simulink model "CaseStudyII_9_Bus"  (R2020a)
settings: Solver=FixedStepAuto  StartTime=0.0  StopTime=Tend  FixedStep=T_s_power  MaxStep=5.0E-5  RelTol=1e-3
values from neighbouring files (symbols this model uses):
  B_s46 = b_s46*Cb    (= 9.5071761847e-07)    [Data_CaseStudyI.m]    (also in Data_CaseStudyII.m; Data_InitialSystem.m)
  B_s54 = b_s54*Cb    (= 1.05902722057e-06)    [Data_CaseStudyI.m]    (also in Data_CaseStudyII.m; Data_InitialSystem.m)
  B_s69 = b_s69*Cb    (= 2.15415764185e-06)    [Data_CaseStudyI.m]    (also in Data_CaseStudyII.m; Data_InitialSystem.m)
  B_s75 = b_s75*Cb    (= 1.84126323577e-06)    [Data_CaseStudyI.m]    (also in Data_CaseStudyII.m; Data_InitialSystem.m)
  B_s87 = b_s87*Cb    (= 8.96562817417e-07)    [Data_CaseStudyI.m]    (also in Data_CaseStudyII.m; Data_InitialSystem.m)
  B_s98 = b_s98*Cb    (= 1.25759482443e-06)    [Data_CaseStudyI.m]    (also in Data_CaseStudyII.m; Data_InitialSystem.m)
  C_dc_DVPP_1_2 = 0.008*(n_DVPP_1_2)    (= 0.8)    [Data_CaseStudyI.m]    (also in Data_CaseStudyII.m)
  C_dc_DVPP_1_3 = 0.008*(n_DVPP_1_3)    (= 0.4)    [Data_CaseStudyI.m]    (also in Data_CaseStudyII.m)
  C_dc_DVPP_3_1 = 0.008*(n_DVPP_3_1)    (= 1.128)    [Data_CaseStudyII.m]
  C_dc_DVPP_3_2 = 0.008*(n_DVPP_3_2)    (= 0.848)    [Data_CaseStudyII.m]
  C_dc_DVPP_3_3 = 0.008*(n_DVPP_3_3)    (= 1.28)    [Data_CaseStudyII.m]
  Dp_DVPP_3_pu = 1/dp_DVPP_3    (= 33.3333333333)    [Data_CaseStudyII.m]
  Dq1_DVPP_3_pu = 100    [Data_CaseStudyII.m]
  fb = 50    [Data_CaseStudyI.m]    (also in Data_CaseStudyII.m; Data_InitialSystem.m)
  HGov_dyn = HGov_delay*H_tr_droop    [Data_CaseStudyI.m]    (also in Data_CaseStudyII.m; Data_InitialSystem.m)
  HTurb_tot = H_water_way    [Data_CaseStudyI.m]    (also in Data_CaseStudyII.m; Data_InitialSystem.m)
  I_m_DVPP_1_2 = 2/3*Sb_DVPP_1_2/V_m_DVPP_1_2    [Data_CaseStudyI.m]    (also in Data_CaseStudyII.m)
  I_m_DVPP_1_3 = 2/3*Sb_DVPP_1_3/V_m_DVPP_1_3    [Data_CaseStudyI.m]    (also in Data_CaseStudyII.m)
  I_m_DVPP_3_1 = 2/3*Sb_DVPP_3_1/V_m_DVPP_3_1    [Data_CaseStudyII.m]
  I_m_DVPP_3_2 = 2/3*Sb_DVPP_3_2/V_m_DVPP_3_2    [Data_CaseStudyII.m]
  I_m_DVPP_3_3 = 2/3*Sb_DVPP_3_3/V_m_DVPP_3_3    [Data_CaseStudyII.m]
  i_star_max = 1.3    [Data_CaseStudyI.m]    (also in Data_CaseStudyII.m)
  iabc_DVPP_1_2_0 = T0*idq0_DVPP_1_2    [Data_CaseStudyI.m]    (also in Data_CaseStudyII.m)
  iabc_DVPP_1_3_0 = T0*idq0_DVPP_1_3    [Data_CaseStudyI.m]    (also in Data_CaseStudyII.m)
  iabc_DVPP_3_1_0 = T0*idq0_DVPP_3_1    [Data_CaseStudyII.m]
  iabc_DVPP_3_2_0 = T0*idq0_DVPP_3_2    [Data_CaseStudyII.m]
  iabc_DVPP_3_3_0 = T0*idq0_DVPP_3_3    [Data_CaseStudyII.m]
  K2_DVPP_1 = [-0.0221795494247 -1.60799665656 0.160449825826 -2.94803557381 -11.8081988371 -9.75170960256 0.00463021906909 -49.1667298155]    [ControlGains_DVPP1.mat]
  K3_DVPP_1 = [-0.0591512752956 -1.61493903379 -27.2946107927 -16.2119211358 -14.3657419818 2.05688388773 -2.27328406162 0.146700393037 -150.920793597]    [ControlGains_DVPP1.mat]
  k_dc_DVPP_1_2 = eta_DVPP_1_2/(Vdc_n_DVPP_1_2*m_p_DVPP_1_2)    [Data_CaseStudyI.m]    (also in Data_CaseStudyII.m)
  k_dc_DVPP_1_3 = eta_DVPP_1_3/(Vdc_n_DVPP_1_3*m_p_DVPP_1_3)    [Data_CaseStudyI.m]    (also in Data_CaseStudyII.m)
  k_dc_DVPP_3_1 = eta_DVPP_3_1/(Vdc_n_DVPP_3_1*m_p_DVPP_3_1)    [Data_CaseStudyII.m]
  k_dc_DVPP_3_2 = eta_DVPP_3_2/(Vdc_n_DVPP_3_2*m_p_DVPP_3_2)    [Data_CaseStudyII.m]
  k_dc_DVPP_3_3 = eta_DVPP_3_3/(Vdc_n_DVPP_3_3*m_p_DVPP_3_3)    [Data_CaseStudyII.m]
  ki_i_pu = 1.19    [Data_CaseStudyI.m]    (also in Data_CaseStudyII.m)
  ki_pll = 1700    [Data_CaseStudyI.m]    (also in Data_CaseStudyII.m)
  ki_q_pu = 0.005    [Data_CaseStudyI.m]    (also in Data_CaseStudyII.m)
  kp_i_pu = 0.73    [Data_CaseStudyI.m]    (also in Data_CaseStudyII.m)
  kp_pll = 150    [Data_CaseStudyI.m]    (also in Data_CaseStudyII.m)
  kp_q_pu = 0.05    [Data_CaseStudyI.m]    (also in Data_CaseStudyII.m)
  L1_DVPP_1_2_pu = 0.0186/m_DVPP_1_2    (= 0.000372)    [Data_CaseStudyI.m]    (also in Data_CaseStudyII.m)
  L1_DVPP_1_3_pu = 0.0186/m_DVPP_1_3    (= 0.000744)    [Data_CaseStudyI.m]    (also in Data_CaseStudyII.m)
  L1_DVPP_3_1_pu = 0.0186/m_DVPP_3_1    (= 0.000263829787234)    [Data_CaseStudyII.m]
  L1_DVPP_3_2_pu = 0.0186/m_DVPP_3_2    (= 0.000350943396226)    [Data_CaseStudyII.m]
  L1_DVPP_3_3_pu = 0.0186/m_DVPP_3_3    (= 0.0002325)    [Data_CaseStudyII.m]
  l1_MVHV1 = 0    [Data_CaseStudyI.m]    (also in Data_CaseStudyII.m; Data_InitialSystem.m)
  l1_MVHV2 = 0    [Data_CaseStudyI.m]    (also in Data_CaseStudyII.m; Data_InitialSystem.m)
  l1_MVHV3 = 0    [Data_CaseStudyI.m]    (also in Data_CaseStudyII.m; Data_InitialSystem.m)
  L2_DVPP_1_2_pu = L1_DVPP_1_2_pu    (= 0.000372)    [Data_CaseStudyI.m]    (also in Data_CaseStudyII.m)
  L2_DVPP_1_3_pu = L1_DVPP_1_3_pu    (= 0.000744)    [Data_CaseStudyI.m]    (also in Data_CaseStudyII.m)
  L2_DVPP_3_1_pu = L1_DVPP_3_1_pu    (= 0.000263829787234)    [Data_CaseStudyII.m]
  L2_DVPP_3_2_pu = L1_DVPP_3_2_pu    (= 0.000350943396226)    [Data_CaseStudyII.m]
  L2_DVPP_3_3_pu = L1_DVPP_3_3_pu    (= 0.0002325)    [Data_CaseStudyII.m]
  l2_MVHV1 = l_s14    (= 0.0576)    [Data_CaseStudyI.m]    (also in Data_CaseStudyII.m; Data_InitialSystem.m)
  l2_MVHV2 = l_s72    (= 0.0625)    [Data_CaseStudyI.m]    (also in Data_CaseStudyII.m; Data_InitialSystem.m)
  l2_MVHV3 = l_s39    (= 0.0586)    [Data_CaseStudyI.m]    (also in Data_CaseStudyII.m; Data_InitialSystem.m)
  l_f_DVPP_1_2 = L_f_DVPP_1_2*w_b/Zb_DVPP_1_2    [Data_CaseStudyI.m]    (also in Data_CaseStudyII.m)
  L_f_DVPP_1_2 = (1/(n_DVPP_1_2))*600*10^-6    (= 6e-06)    [Data_CaseStudyI.m]    (also in Data_CaseStudyII.m)
  l_f_DVPP_1_3 = L_f_DVPP_1_3*w_b/Zb_DVPP_1_3    [Data_CaseStudyI.m]    (also in Data_CaseStudyII.m)
  L_f_DVPP_1_3 = (1/(n_DVPP_1_3))*600*10^-6    (= 1.2e-05)    [Data_CaseStudyI.m]    (also in Data_CaseStudyII.m)
  l_f_DVPP_3_1 = L_f_DVPP_3_1*w_b/Zb_DVPP_3_1    [Data_CaseStudyII.m]
  L_f_DVPP_3_1 = (1/(n_DVPP_3_1))*600*10^-6    (= 4.25531914894e-06)    [Data_CaseStudyII.m]
  l_f_DVPP_3_2 = L_f_DVPP_3_2*w_b/Zb_DVPP_3_2    [Data_CaseStudyII.m]
  L_f_DVPP_3_2 = (1/(n_DVPP_3_2))*600*10^-6    (= 5.66037735849e-06)    [Data_CaseStudyII.m]
  l_f_DVPP_3_3 = L_f_DVPP_3_3*w_b/Zb_DVPP_3_3    [Data_CaseStudyII.m]
  L_f_DVPP_3_3 = (1/(n_DVPP_3_3))*600*10^-6    (= 3.75e-06)    [Data_CaseStudyII.m]
  L_s46 = l_s46*Lb    (= 0.154915055408)    [Data_CaseStudyI.m]    (also in Data_CaseStudyII.m; Data_InitialSystem.m)
  L_s54 = l_s54*Lb    (= 0.143128040323)    [Data_CaseStudyI.m]    (also in Data_CaseStudyII.m; Data_InitialSystem.m)
  L_s69 = l_s69*Lb    (= 0.286256080645)    [Data_CaseStudyI.m]    (also in Data_CaseStudyII.m; Data_InitialSystem.m)
  L_s75 = l_s75*Lb    (= 0.271101346964)    [Data_CaseStudyI.m]    (also in Data_CaseStudyII.m; Data_InitialSystem.m)
  L_s87 = l_s87*Lb    (= 0.12123786945)    [Data_CaseStudyI.m]    (also in Data_CaseStudyII.m; Data_InitialSystem.m)
  L_s98 = l_s98*Lb    (= 0.16973301723)    [Data_CaseStudyI.m]    (also in Data_CaseStudyII.m; Data_InitialSystem.m)
  LPV_K1_DVPP_3 = [0.014519129833 -1.24253756746e-17 -0.00331576987938 -1.41950397655e-17 -0.00331577010739 -1.6423216922e-19 0.0145191298795 1.47256053017e-18 1.92456501739e-17 0.00968260817745 7.5102914291e-19 0.0096826081765 ... (80 elements, 8x10)]    [ControlGains_DVPP3_LPV.mat]
  LPV_K2_DVPP_3 = [0.0299413265511 -2.72480441208e-16 -0.00563144274341 -6.63344905835e-17 -0.00563144273182 -1.08918556426e-16 0.0299413268326 -1.32404731664e-16 -4.78559537004e-17 -0.00914230292149 -8.50409089014e-21 -0.00914230292147 ... (80 elements, 8x10)]    [ControlGains_DVPP3_LPV.mat]
  LPV_K3_DVPP_3 = [-0.0173301370849 5.00398589077e-17 -0.0636125194304 3.31757376688e-17 -0.0636125164794 5.41726806116e-17 -0.017330137145 2.43427565927e-17 -0.0400570975704 -5.68753124238e-17 -0.0574012283733 2.45717741258e-17 ... (192 elements, 16x12)]    [ControlGains_DVPP3_LPV.mat]
  Mp_DVPP_3_pu = 13    [Data_CaseStudyII.m]
  P_L = pL*Sb    (= 300000000)    [Data_CaseStudyI.m]    (also in Data_CaseStudyII.m; Data_InitialSystem.m)
  p_set_bus1 = P_set_bus1/SbSG1    (= 0.731707317073)    [Data_CaseStudyI.m]    (also in Data_CaseStudyII.m; Data_InitialSystem.m)
  p_set_bus2 = P_set_bus2/SbSG2    (= 0.756707317073)    [Data_CaseStudyI.m]    (also in Data_CaseStudyII.m; Data_InitialSystem.m)
  Pb_DVPP_3_1 = 37e6    (= 37000000)    [Data_CaseStudyII.m]
  Pb_DVPP_3_2 = 28e6    (= 28000000)    [Data_CaseStudyII.m]
  Pb_DVPP_3_3 = 0e6    (= 0)    [Data_CaseStudyII.m]
  pset_DVPP_1_1 = P_set_bus1/SbSG1    (= 0.731707317073)    [Data_CaseStudyI.m]    (also in Data_CaseStudyII.m)
  pset_DVPP_1_2 = 0    [Data_CaseStudyI.m]    (also in Data_CaseStudyII.m)
  pset_DVPP_1_3 = 0    [Data_CaseStudyI.m]    (also in Data_CaseStudyII.m)
  pset_DVPP_3_1 = (0.6*P_set_bus3)/Sb_DVPP_3_1    (= 0.398546964193)    [Data_CaseStudyII.m]
  pset_DVPP_3_2 = (0.4*P_set_bus3)/Sb_DVPP_3_2    (= 0.353428439945)    [Data_CaseStudyII.m]
  pset_DVPP_3_3 = 0    [Data_CaseStudyII.m]
  Q_L = qL*Sb    (= 82500000)    [Data_CaseStudyI.m]    (also in Data_CaseStudyII.m; Data_InitialSystem.m)
  qset_DVPP_1_2 = 0    [Data_CaseStudyI.m]    (also in Data_CaseStudyII.m)
  qset_DVPP_1_3 = 0    [Data_CaseStudyI.m]    (also in Data_CaseStudyII.m)
  qset_DVPP_3_1 = 0    [Data_CaseStudyII.m]
  qset_DVPP_3_2 = 0    [Data_CaseStudyII.m]
  qset_DVPP_3_3 = 0    [Data_CaseStudyII.m]
  R1_DVPP_1_2_pu = 0.00734/m_DVPP_1_2    (= 0.0001468)    [Data_CaseStudyI.m]    (also in Data_CaseStudyII.m)
  R1_DVPP_1_3_pu = 0.00734/m_DVPP_1_3    (= 0.0002936)    [Data_CaseStudyI.m]    (also in Data_CaseStudyII.m)
  R1_DVPP_3_1_pu = 0.00734/m_DVPP_3_1    (= 0.000104113475177)    [Data_CaseStudyII.m]
  R1_DVPP_3_2_pu = 0.00734/m_DVPP_3_2    (= 0.000138490566038)    [Data_CaseStudyII.m]
  R1_DVPP_3_3_pu = 0.00734/m_DVPP_3_3    (= 9.175e-05)    [Data_CaseStudyII.m]
  r1_MVHV1 = 1e-6    (= 1e-06)    [Data_CaseStudyI.m]    (also in Data_CaseStudyII.m; Data_InitialSystem.m)
  r1_MVHV2 = 1e-6    (= 1e-06)    [Data_CaseStudyI.m]    (also in Data_CaseStudyII.m; Data_InitialSystem.m)
  r1_MVHV3 = 1e-6    (= 1e-06)    [Data_CaseStudyI.m]    (also in Data_CaseStudyII.m; Data_InitialSystem.m)
  R2_DVPP_1_2_pu = R1_DVPP_1_2_pu    (= 0.0001468)    [Data_CaseStudyI.m]    (also in Data_CaseStudyII.m)
  R2_DVPP_1_3_pu = R1_DVPP_1_3_pu    (= 0.0002936)    [Data_CaseStudyI.m]    (also in Data_CaseStudyII.m)
  R2_DVPP_3_1_pu = R1_DVPP_3_1_pu    (= 0.000104113475177)    [Data_CaseStudyII.m]
  R2_DVPP_3_2_pu = R1_DVPP_3_2_pu    (= 0.000138490566038)    [Data_CaseStudyII.m]
  R2_DVPP_3_3_pu = R1_DVPP_3_3_pu    (= 9.175e-05)    [Data_CaseStudyII.m]
  r2_MVHV1 = 1e-6    (= 1e-06)    [Data_CaseStudyI.m]    (also in Data_CaseStudyII.m; Data_InitialSystem.m)
  r2_MVHV2 = 1e-6    (= 1e-06)    [Data_CaseStudyI.m]    (also in Data_CaseStudyII.m; Data_InitialSystem.m)
  r2_MVHV3 = 1e-6    (= 1e-06)    [Data_CaseStudyI.m]    (also in Data_CaseStudyII.m; Data_InitialSystem.m)
  R_dc_DVPP_1_2 = (Vdc_n_DVPP_1_2/(0.05*(Sb_DVPP_1_2)/Vdc_n_DVPP_1_2))    [Data_CaseStudyI.m]    (also in Data_CaseStudyII.m)
  R_dc_DVPP_1_3 = (Vdc_n_DVPP_1_3/(0.05*(Sb_DVPP_1_3)/Vdc_n_DVPP_1_3))    [Data_CaseStudyI.m]    (also in Data_CaseStudyII.m)
  R_dc_DVPP_3_1 = (Vdc_n_DVPP_3_1/(0.05*(Sb_DVPP_3_1)/Vdc_n_DVPP_3_1))    [Data_CaseStudyII.m]
  R_dc_DVPP_3_2 = (Vdc_n_DVPP_3_2/(0.05*(Sb_DVPP_3_2)/Vdc_n_DVPP_3_2))    [Data_CaseStudyII.m]
  R_dc_DVPP_3_3 = (Vdc_n_DVPP_3_3/(0.05*(Sb_DVPP_3_3)/Vdc_n_DVPP_3_3))    [Data_CaseStudyII.m]
  r_f_DVPP_1_2 = R_f_DVPP_1_2/Zb_DVPP_1_2    [Data_CaseStudyI.m]    (also in Data_CaseStudyII.m)
  R_f_DVPP_1_2 = 0.02/n_DVPP_1_2    (= 0.0002)    [Data_CaseStudyI.m]    (also in Data_CaseStudyII.m)
  r_f_DVPP_1_3 = R_f_DVPP_1_3/Zb_DVPP_1_3    [Data_CaseStudyI.m]    (also in Data_CaseStudyII.m)
  R_f_DVPP_1_3 = 0.02/n_DVPP_1_3    (= 0.0004)    [Data_CaseStudyI.m]    (also in Data_CaseStudyII.m)
  r_f_DVPP_3_1 = R_f_DVPP_3_1/Zb_DVPP_3_1    [Data_CaseStudyII.m]
  ... (+104 more)
undefined symbols (not defined in the file or in its folder): A, B, C, Continuous, Dd, Efd0, gcbh, i_dc, Ka, Kf, p2set, SbSM2, sps_rtmsupport, spsST1AModel, Ta, Tb, Tb1, Tc, Tc1, Tf, VA0, VAmax, VAmin, VImax, VImin, VRmax, VRmin
libraries: powerlib x95, powerlib_meascontrol x41, cstblocks x15, sps_avr x1, simulink_extras x1, simulink x1
(part 2 of 5)

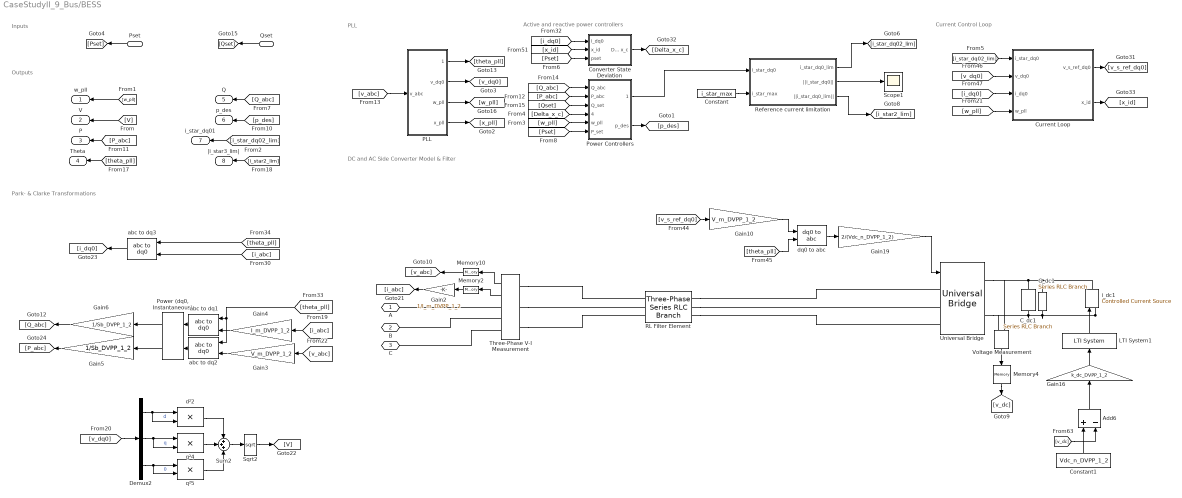
== system CaseStudyII_9_Bus/BESS ==
  note: Inputs
  note: Active and reactive power controllers
  note: PLL
  note: Outputs
  note: Current Control Loop
  note: Park- & Clarke Transformations
  note: DC and AC Side Converter Model & Filter
  Qset : Inport
  Pset : Inport  Port=2
  Add6 : Sum  Inputs=+-
  C_dc1 : powerlib/Elements/Series RLC Branch  LConnTagsString=__new0  RConnTagsString=__new0  BranchType=C  Resistance=1  Inductance=1e-3  SetiL0=off  InitialCurrent=0  Capacitance=C_dc_DVPP_1_2  Setx0=off  InitialVoltage=Vdc_n  Measurements=None
  Constant : Constant  Value=i_star_max
  Constant1 : Constant  Value=Vdc_n_DVPP_1_2
  Converter State Deviation : Subsystem
  Current Loop : Subsystem  AncestorBlock=Library/Grid-Forming Converter Controlled by Droop Control /Current Loop
  Demux2 : Demux  Outputs=3
  G_dc1 : powerlib/Elements/Series RLC Branch  LConnTagsString=__new0  RConnTagsString=__new0  BranchType=R  Resistance=R_dc_DVPP_1_2  Inductance=1e-3  SetiL0=off  InitialCurrent=0  Capacitance=1e-6  Setx0=off  InitialVoltage=0  Measurements=None
  Gain10 : Gain  Gain=V_m_DVPP_1_2
  Gain16 : Gain  Gain=k_dc_DVPP_1_2
  Gain19 : Gain  Gain=2/(Vdc_n_DVPP_1_2)
  Gain2 : Gain  Gain=1/I_m_DVPP_1_2
  Gain3 : Gain  Gain=V_m_DVPP_1_2
  Gain4 : Gain  Gain=I_m_DVPP_1_2
  Gain5 : Gain  Gain=1/Sb_DVPP_1_2
  Gain6 : Gain  Gain=1/Sb_DVPP_1_2
  LTI System1 : cstblocks/LTI System  sys=tf(1,[tau_dc_DVPP_1_2 1])  IC=[]
  Memory10 : Memory  InitialCondition=[vabc_DVPP_1_2_0_pu(1), vabc_DVPP_1_2_0_pu(2), vabc_DVPP_1_2_0_pu(3)]
  Memory2 : Memory  InitialCondition=[iabc_DVPP_1_2_0(1), iabc_DVPP_1_2_0(2), iabc_DVPP_1_2_0(3)]
  Memory4 : Memory
  PLL : Subsystem
  "Power (dq0, Instantaneous)" : powerlib_meascontrol/Measurements/Power (dq0, Instantaneous)
      settings: SourceProductBaseCode=PS
  Power Controllers : Subsystem
  RL Filter Element : powerlib/Elements/Three-Phase Series RLC Branch  LConnTagsString=A|B|C  RConnTagsString=A|B|C  BranchType=RL  Resistance=R_f_DVPP_1_2  Inductance=L_f_DVPP_1_2  Capacitance=0  Measurements=Branch currents
  Reference current limitation : Subsystem
  Scope1 : Scope
  Sqrt2 : Sqrt  SaturateOnIntegerOverflow=on
  Sum2 : Sum  Inputs=+++  InputSameDT=on  SaturateOnIntegerOverflow=on  OutDataTypeStr=Inherit: Same as first input
  Three-Phase V-I Measurement : powerlib/Measurements/Three-Phase V-I Measurement  VoltageMeasurement=phase-to-ground  SetLabelV=off  LabelV=Vabc  Vpu=on  VpuLL=off  CurrentMeasurement=yes  SetLabelI=off  LabelI=Iabc  Ipu=off  Pbase=Sb_conv  Vbase=VbLV_DVPP_1_2  OutputType=Complex  PhasorSimulation=off  PSBequivalent=0
  Universal Bridge : powerlib/Power Electronics/Universal Bridge  Arms=3  SnubberResistance=1e5  SnubberCapacitance=inf  Device=Average-model based VSC  Ron=1e-3  Lon=0  ForwardVoltages="[  0  0  ]"  ForwardVoltage=0  GTOparameters=[ 10e-6 , 20e-6 ]  IGBTparameters=[ 1e-6 , 2e-6 ]  Measurements=None  Measurements_2=None  converterType=Rectifier
  Voltage Measurement : powerlib/Measurements/Voltage Measurement  PhasorSimulation=off  OutputType=Complex  PSBequivalent=0
  abc to dq1 : powerlib_meascontrol/Transformations/abc to dq0  Alignment=90 degrees behind phase A axis
  abc to dq2 : powerlib_meascontrol/Transformations/abc to dq0  Alignment=90 degrees behind phase A axis
  abc to dq3 : powerlib_meascontrol/Transformations/abc to dq0  Alignment=90 degrees behind phase A axis
  dq0 to abc : powerlib_meascontrol/Transformations/dq0 to abc  Alignment=90 degrees behind phase A axis
  d²2 : Product  InputSameDT=on  RndMeth=Zero  SaturateOnIntegerOverflow=on  OutDataTypeStr=Inherit: Same as first input
  i_dc1 : powerlib/Electrical Sources/Controlled Current Source  Initialize=off  Source_Type=DC  Amplitude=i_dc  Phase=0  Frequency=0  Measurements=None
  q²4 : Product  InputSameDT=on  RndMeth=Zero  SaturateOnIntegerOverflow=on  OutDataTypeStr=Inherit: Same as first input
  q²5 : Product  InputSameDT=on  RndMeth=Zero  SaturateOnIntegerOverflow=on  OutDataTypeStr=Inherit: Same as first input
  A : PMIOPort  Side=Right
  B : PMIOPort  Port=2  Side=Right
  C : PMIOPort  Port=3  Side=Right
  w_pll : Outport  VectorParamsAs1DForOutWhenUnconnected=off
  V : Outport  Port=2  VectorParamsAs1DForOutWhenUnconnected=off
  P : Outport  Port=3  VectorParamsAs1DForOutWhenUnconnected=off
  Theta : Outport  Port=4  VectorParamsAs1DForOutWhenUnconnected=off
  Q : Outport  Port=5  VectorParamsAs1DForOutWhenUnconnected=off
  p_des : Outport  Port=6  VectorParamsAs1DForOutWhenUnconnected=off
  i_star_dq01 : Outport  Port=7  VectorParamsAs1DForOutWhenUnconnected=off
  |i_star3_lim| : Outport  Port=8  VectorParamsAs1DForOutWhenUnconnected=off
  wires:
  PLL/4(x_pll) -> [x_pll]
  [v_abc] -> PLL/1(v_abc)
  [i_star_dq02_lim] -> i_star_dq01/1
  PLL/2(v_dq0) -> [v_dq0]
  [p_des] -> p_des/1
  PLL/1(theta_pll) -> [theta_pll]
  PLL/3(w_pll) -> [w_pll]
  [V] -> V/1
  [w_pll] -> w_pll/1
  [theta_pll] -> Theta/1
  Power Controllers/2(p_des) -> [p_des]
  Power Controllers/1(i_star_dq0) -> Reference current limitation/1(i_star_dq0)
  [Q_abc] -> Q/1
  Qset/1 -> [Qset]
  [P_abc] -> P/1
  Constant/1 -> Reference current limitation/2(i_star_max)
  Reference current limitation/2(||i_star_dq0||) -> Scope1/1
  [i_star2_lim] -> |i_star3_lim|/1
  [w_pll] -> Current Loop/4(w_pll)
  [i_dq0] -> Current Loop/3(i_dq0)
  Reference current limitation/1(i_star_dq0_lim) -> [i_star_dq02_lim]
  [v_dq0] -> Current Loop/2(v_dq0)
  [v_dq0] -> Demux2/1
  Sum2/1 -> Sqrt2/1
  [i_abc] -> Gain4/1
  Demux2/3 -> q²5/2, q²5/1  "0"
  Demux2/1 -> d²2/1, d²2/2  "d"
  abc to dq1/1 -> "Power (dq0, Instantaneous)"/2
  Three-Phase V-I Measurement/1 -> Memory10/1
  Gain5/1 -> [P_abc]
  Gain4/1 -> abc to dq1/1
  Gain3/1 -> abc to dq2/1
  q²4/1 -> Sum2/2
  Gain6/1 -> [Q_abc]
  Gain19/1 -> Universal Bridge/1
  Add6/1 -> Gain16/1
  [v_abc] -> Gain3/1
  [theta_pll] -> abc to dq3/2
  abc to dq3/1 -> [i_dq0]
  Voltage Measurement/1 -> Memory4/1
  d²2/1 -> Sum2/1
  [theta_pll] -> abc to dq2/2, abc to dq1/2
  dq0 to abc/1 -> Gain19/1
  Memory10/1 -> [v_abc]
  "Power (dq0, Instantaneous)"/2 -> Gain6/1
  Sqrt2/1 -> [V]
  "Power (dq0, Instantaneous)"/1 -> Gain5/1
  Demux2/2 -> q²4/1, q²4/2  "q"
  [v_dc] -> Add6/2
  q²5/1 -> Sum2/3
  abc to dq2/1 -> "Power (dq0, Instantaneous)"/1
  Memory4/1 -> [v_dc]
  LTI System1/1 -> i_dc1/1
  Gain10/1 -> dq0 to abc/1
  [theta_pll] -> dq0 to abc/2
  [i_abc] -> abc to dq3/1
  [v_s_ref_dq0] -> Gain10/1
  Gain16/1 -> LTI System1/1
  Constant1/1 -> Add6/1
  Converter State Deviation/1(Delta x_c) -> [Delta_x_c]
  Current Loop/2(x_id) -> [x_id]
  Current Loop/1(v_s_ref_dq0) -> [v_s_ref_dq0]
  [P_abc] -> Power Controllers/2(P_abc)
  [Delta_x_c] -> Power Controllers/4(Delta x_c)
  [Q_abc] -> Power Controllers/1(Q_abc)
  [Qset] -> Power Controllers/3(Q_set)
  [x_id] -> Converter State Deviation/2(x_id)
  [i_dq0] -> Converter State Deviation/1(i_dq0)
  Reference current limitation/3(||i_star_dq0_lim||) -> [i_star2_lim]
  [i_star_dq02_lim] -> Current Loop/1(i_star_dq0)
  [w_pll] -> Power Controllers/5(w_pll)
  [Pset] -> Converter State Deviation/3(pset)
  Pset/1 -> [Pset]
  [Pset] -> Power Controllers/6(P_set)
  Gain2/1 -> [i_abc]
  Memory2/1 -> Gain2/1
  Three-Phase V-I Measurement/2 -> Memory2/1
  connections:
  i_dc1/LConn1 -- G_dc1/RConn1 -- Voltage Measurement/LConn2 -- Universal Bridge/RConn2 -- C_dc1/RConn1
  i_dc1/RConn1 -- G_dc1/LConn1 -- Voltage Measurement/LConn1 -- Universal Bridge/RConn1 -- C_dc1/LConn1
  RL Filter Element/RConn3 -- Universal Bridge/LConn3
  RL Filter Element/RConn2 -- Universal Bridge/LConn2
  RL Filter Element/RConn1 -- Universal Bridge/LConn1
  Three-Phase V-I Measurement/LConn1 -- RL Filter Element/LConn1
  Three-Phase V-I Measurement/LConn2 -- RL Filter Element/LConn2
  Three-Phase V-I Measurement/LConn3 -- RL Filter Element/LConn3
  Three-Phase V-I Measurement/RConn1 -- A/RConn1
  Three-Phase V-I Measurement/RConn2 -- B/RConn1
  Three-Phase V-I Measurement/RConn3 -- C/RConn1

== system CaseStudyII_9_Bus/DVPP Operator  ==
  pmax_1 : Inport
  pmax_2 : Inport  Port=2
  Add : Sum
  Constant : Constant  Value=Sb_DVPP_3_1
  Constant1 : Constant  Value=Sb_DVPP_3_2
  Constant2 : Constant  Value=Sb_DVPP_3_3
  Constant3 : Constant  Value=Pb_DVPP_3_3
  Divide : Product  Inputs=*/
  Divide1 : Product  Inputs=/*
  MATLAB Function : MATLAB Function  TreatAsAtomicUnit=on
  theta1_p : Outport
  theta2_p : Outport  Port=2
  theta1_q : Outport  Port=3
  theta2_q : Outport  Port=4
  theta3_q : Outport  Port=5
  wires:
  pmax_2/1 -> Add/2, MATLAB Function/5(P2), Divide1/2
  pmax_1/1 -> Divide/1, MATLAB Function/4(P1), Add/1
  Add/1 -> Divide1/1, Divide/2
  Divide1/1 -> theta2_p/1
  Divide/1 -> theta1_p/1
  Constant/1 -> MATLAB Function/1(S1)
  Constant1/1 -> MATLAB Function/2(S2)
  Constant2/1 -> MATLAB Function/3(S3)
  Constant3/1 -> MATLAB Function/6(P3)
  MATLAB Function/1(theta1_q) -> theta1_q/1
  MATLAB Function/2(theta2_q) -> theta2_q/1
  MATLAB Function/3(theta3_q) -> theta3_q/1

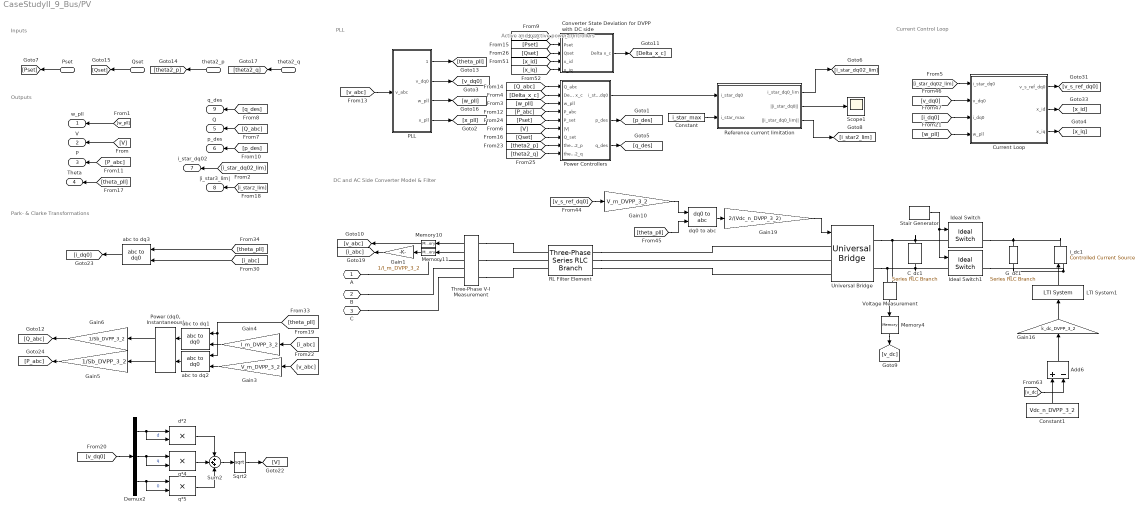
== system CaseStudyII_9_Bus/PV ==
  note: PLL
  note: Park- & Clarke Transformations
  note: Outputs
  note: Active and reactive power controllers
  note: Current Control Loop
  note: DC and AC Side Converter Model & Filter
  note: Inputs
  Pset : Inport
  Qset : Inport  Port=2
  theta2_p : Inport  Port=3
  theta2_q : Inport  Port=4
  Add6 : Sum  Inputs=+-
  C_dc1 : powerlib/Elements/Series RLC Branch  LConnTagsString=__new0  RConnTagsString=__new0  BranchType=C  Resistance=1  Inductance=1e-3  SetiL0=off  InitialCurrent=0  Capacitance=C_dc_DVPP_3_2  Setx0=off  InitialVoltage=Vdc_n  Measurements=None
  Constant : Constant  Value=i_star_max
  Constant1 : Constant  Value=Vdc_n_DVPP_3_2
  Converter State Deviation for DVPP with DC side : Subsystem
  Current Loop : Subsystem  AncestorBlock=Library/Grid-Forming Converter Controlled by Droop Control /Current Loop
  Demux2 : Demux  Outputs=3
  G_dc1 : powerlib/Elements/Series RLC Branch  LConnTagsString=__new0  RConnTagsString=__new0  BranchType=R  Resistance=R_dc_DVPP_3_2  Inductance=1e-3  SetiL0=off  InitialCurrent=0  Capacitance=1e-6  Setx0=off  InitialVoltage=0  Measurements=None
  Gain1 : Gain  Gain=1/I_m_DVPP_3_2
  Gain10 : Gain  Gain=V_m_DVPP_3_2
  Gain16 : Gain  Gain=k_dc_DVPP_3_2
  Gain19 : Gain  Gain=2/(Vdc_n_DVPP_3_2)
  Gain3 : Gain  Gain=V_m_DVPP_3_2
  Gain4 : Gain  Gain=I_m_DVPP_3_2
  Gain5 : Gain  Gain=1/Sb_DVPP_3_2
  Gain6 : Gain  Gain=1/Sb_DVPP_3_2
  Ideal Switch : powerlib/Power Electronics/Ideal Switch  Ron=0.001  Lon=0  IC=1  Rs=1e10  Cs=Inf  Measurements=on
  Ideal Switch1 : powerlib/Power Electronics/Ideal Switch  Ron=0.001  Lon=0  IC=1  Rs=1e10  Cs=Inf  Measurements=on
  LTI System1 : cstblocks/LTI System  sys=tf(1,[tau_dc_DVPP_3_2 1])  IC=[]
  Memory10 : Memory  InitialCondition=[vabc_DVPP_3_2_0_pu(1), vabc_DVPP_3_2_0_pu(2), vabc_DVPP_3_2_0_pu(3)]
  Memory11 : Memory  InitialCondition=[iabc_DVPP_3_2_0(1), iabc_DVPP_3_2_0(2), iabc_DVPP_3_2_0(3)]
  Memory4 : Memory
  PLL : Subsystem
  "Power (dq0, Instantaneous)" : powerlib_meascontrol/Measurements/Power (dq0, Instantaneous)
      settings: SourceProductBaseCode=PS
  Power Controllers : Subsystem
  RL Filter Element : powerlib/Elements/Three-Phase Series RLC Branch  LConnTagsString=A|B|C  RConnTagsString=A|B|C  BranchType=RL  Resistance=R_f_DVPP_3_2  Inductance=L_f_DVPP_3_2  Capacitance=0  Measurements=Branch currents
  Reference current limitation : Subsystem
  Scope1 : Scope
  Sqrt2 : Sqrt  SaturateOnIntegerOverflow=on
  Stair Generator : powerlib_meascontrol/Pulse & Signal Generators/Stair Generator  t=[0 T_cloud]  e=[1 0]  Ts=0
      settings: SourceProductBaseCode=MT,PS
  Sum2 : Sum  Inputs=+++  InputSameDT=on  SaturateOnIntegerOverflow=on  OutDataTypeStr=Inherit: Same as first input
  Three-Phase V-I Measurement : powerlib/Measurements/Three-Phase V-I Measurement  VoltageMeasurement=phase-to-ground  SetLabelV=off  LabelV=Vabc  Vpu=on  VpuLL=off  CurrentMeasurement=yes  SetLabelI=off  LabelI=Iabc  Ipu=off  Pbase=Sb_conv  Vbase=VbLV_DVPP_3_2  OutputType=Complex  PhasorSimulation=off  PSBequivalent=0
  Universal Bridge : powerlib/Power Electronics/Universal Bridge  Arms=3  SnubberResistance=1e5  SnubberCapacitance=inf  Device=Average-model based VSC  Ron=1e-3  Lon=0  ForwardVoltages="[  0  0  ]"  ForwardVoltage=0  GTOparameters=[ 10e-6 , 20e-6 ]  IGBTparameters=[ 1e-6 , 2e-6 ]  Measurements=None  Measurements_2=None  converterType=Rectifier
  Voltage Measurement : powerlib/Measurements/Voltage Measurement  PhasorSimulation=off  OutputType=Complex  PSBequivalent=0
  abc to dq1 : powerlib_meascontrol/Transformations/abc to dq0  Alignment=90 degrees behind phase A axis
  abc to dq2 : powerlib_meascontrol/Transformations/abc to dq0  Alignment=90 degrees behind phase A axis
  abc to dq3 : powerlib_meascontrol/Transformations/abc to dq0  Alignment=90 degrees behind phase A axis
  dq0 to abc : powerlib_meascontrol/Transformations/dq0 to abc  Alignment=90 degrees behind phase A axis
  d²2 : Product  InputSameDT=on  RndMeth=Zero  SaturateOnIntegerOverflow=on  OutDataTypeStr=Inherit: Same as first input
  i_dc1 : powerlib/Electrical Sources/Controlled Current Source  Initialize=off  Source_Type=DC  Amplitude=i_dc  Phase=0  Frequency=0  Measurements=None
  q²4 : Product  InputSameDT=on  RndMeth=Zero  SaturateOnIntegerOverflow=on  OutDataTypeStr=Inherit: Same as first input
  q²5 : Product  InputSameDT=on  RndMeth=Zero  SaturateOnIntegerOverflow=on  OutDataTypeStr=Inherit: Same as first input
  A : PMIOPort  Side=Right
  B : PMIOPort  Port=2  Side=Right
  C : PMIOPort  Port=3  Side=Right
  w_pll : Outport  VectorParamsAs1DForOutWhenUnconnected=off
  V : Outport  Port=2  VectorParamsAs1DForOutWhenUnconnected=off
  P : Outport  Port=3  VectorParamsAs1DForOutWhenUnconnected=off
  Theta : Outport  Port=4  VectorParamsAs1DForOutWhenUnconnected=off
  Q : Outport  Port=5  VectorParamsAs1DForOutWhenUnconnected=off
  p_des : Outport  Port=6  VectorParamsAs1DForOutWhenUnconnected=off
  i_star_dq02 : Outport  Port=7  VectorParamsAs1DForOutWhenUnconnected=off
  |i_star3_lim| : Outport  Port=8  VectorParamsAs1DForOutWhenUnconnected=off
  q_des : Outport  Port=9  VectorParamsAs1DForOutWhenUnconnected=off
  wires:
  [q_des] -> q_des/1
  [v_s_ref_dq0] -> Gain10/1
  Reference current limitation/3(||i_star_dq0_lim||) -> [i_star2_lim]
  [v_dq0] -> Demux2/1
  Three-Phase V-I Measurement/1 -> Memory10/1
  Voltage Measurement/1 -> Memory4/1
  [theta_pll] -> Theta/1
  [P_abc] -> P/1
  Memory11/1 -> Gain1/1
  [i_star_dq02_lim] -> Current Loop/1(i_star_dq0)
  Power Controllers/3(q_des) -> [q_des]
  Current Loop/3(x_iq) -> [x_iq]
  [Delta_x_c] -> Power Controllers/2(Delta x_c)
  Memory4/1 -> [v_dc]
  [v_dq0] -> Current Loop/2(v_dq0)
  Power Controllers/1(i_star_dq0) -> Reference current limitation/1(i_star_dq0)
  [V] -> V/1
  [w_pll] -> w_pll/1
  Current Loop/2(x_id) -> [x_id]
  [i_dq0] -> Current Loop/3(i_dq0)
  Gain1/1 -> [i_abc]
  [i_abc] -> Gain4/1
  PLL/1(theta_pll) -> [theta_pll]
  [v_abc] -> Gain3/1
  Gain5/1 -> [P_abc]
  Gain6/1 -> [Q_abc]
  Sum2/1 -> Sqrt2/1
  d²2/1 -> Sum2/1
  Gain10/1 -> dq0 to abc/1
  [i_star_dq02_lim] -> i_star_dq02/1
  Demux2/3 -> q²5/2, q²5/1  "0"
  dq0 to abc/1 -> Gain19/1
  q²5/1 -> Sum2/3
  LTI System1/1 -> i_dc1/1
  Add6/1 -> Gain16/1
  [i_star2_lim] -> |i_star3_lim|/1
  [Q_abc] -> Power Controllers/1(Q_abc)
  "Power (dq0, Instantaneous)"/2 -> Gain6/1
  [v_dc] -> Add6/2
  abc to dq2/1 -> "Power (dq0, Instantaneous)"/1
  [V] -> Power Controllers/6(|V|)
  "Power (dq0, Instantaneous)"/1 -> Gain5/1
  [i_abc] -> abc to dq3/1
  [theta_pll] -> abc to dq2/2, abc to dq1/2
  Gain16/1 -> LTI System1/1
  [theta_pll] -> dq0 to abc/2
  Sqrt2/1 -> [V]
  [v_abc] -> PLL/1(v_abc)
  [w_pll] -> Current Loop/4(w_pll)
  abc to dq3/1 -> [i_dq0]
  Constant1/1 -> Add6/1
  Gain19/1 -> Universal Bridge/1
  [Q_abc] -> Q/1
  Current Loop/1(v_s_ref_dq0) -> [v_s_ref_dq0]
  [theta_pll] -> abc to dq3/2
  [P_abc] -> Power Controllers/4(P_abc)
  Demux2/1 -> d²2/1, d²2/2  "d"
  Reference current limitation/1(i_star_dq0_lim) -> [i_star_dq02_lim]
  Reference current limitation/2(||i_star_dq0||) -> Scope1/1
  Gain3/1 -> abc to dq2/1
  Constant/1 -> Reference current limitation/2(i_star_max)
  abc to dq1/1 -> "Power (dq0, Instantaneous)"/2
  Demux2/2 -> q²4/1, q²4/2  "q"
  q²4/1 -> Sum2/2
  PLL/4(x_pll) -> [x_pll]
  PLL/2(v_dq0) -> [v_dq0]
  PLL/3(w_pll) -> [w_pll]
  Gain4/1 -> abc to dq1/1
  Memory10/1 -> [v_abc]
  Three-Phase V-I Measurement/2 -> Memory11/1
  [Pset] -> Power Controllers/5(P_set)
  Power Controllers/2(p_des) -> [p_des]
  [p_des] -> p_des/1
  [w_pll] -> Power Controllers/3(w_pll)
  Converter State Deviation for DVPP with DC side/1(Delta x_c) -> [Delta_x_c]
  [x_id] -> Converter State Deviation for DVPP with DC side/4(x_id)
  [x_iq] -> Converter State Deviation for DVPP with DC side/5(x_iq)
  [Qset] -> Converter State Deviation for DVPP with DC side/3(Qset)
  [Pset] -> Converter State Deviation for DVPP with DC side/2(Pset)
  [i_dq0] -> Converter State Deviation for DVPP with DC side/1(i_dq0)
  [Qset] -> Power Controllers/7(Q_set)
  Qset/1 -> [Qset]
  theta2_q/1 -> [theta2_q]
  Pset/1 -> [Pset]
  theta2_p/1 -> [theta2_p]
  [theta2_p] -> Power Controllers/8(theta2_p)
  [theta2_q] -> Power Controllers/9(theta2_q)
  Stair Generator/1 -> Ideal Switch1/1, Ideal Switch/1
  connections:
  i_dc1/RConn1 -- G_dc1/LConn1 -- Ideal Switch/RConn1
  i_dc1/LConn1 -- Ideal Switch1/RConn1 -- G_dc1/RConn1
  B/RConn1 -- Three-Phase V-I Measurement/RConn2
  Three-Phase V-I Measurement/LConn3 -- RL Filter Element/LConn3
  RL Filter Element/RConn1 -- Universal Bridge/LConn1
  Three-Phase V-I Measurement/LConn1 -- RL Filter Element/LConn1
  RL Filter Element/RConn2 -- Universal Bridge/LConn2
  A/RConn1 -- Three-Phase V-I Measurement/RConn1
  C/RConn1 -- Three-Phase V-I Measurement/RConn3
  Three-Phase V-I Measurement/LConn2 -- RL Filter Element/LConn2
  RL Filter Element/RConn3 -- Universal Bridge/LConn3
  Universal Bridge/RConn2 -- Ideal Switch1/LConn1 -- C_dc1/RConn1 -- Voltage Measurement/LConn2
  Voltage Measurement/LConn1 -- Universal Bridge/RConn1 -- C_dc1/LConn1 -- Ideal Switch/LConn1

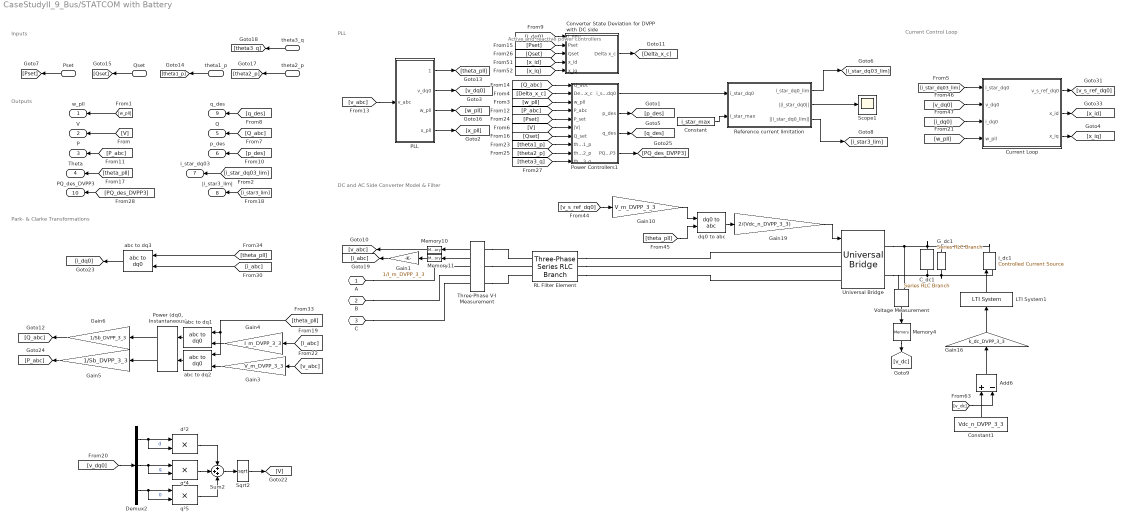
== system CaseStudyII_9_Bus/STATCOM with Battery ==
  note: Current Control Loop
  note: Park- & Clarke Transformations
  note: Outputs
  note: DC and AC Side Converter Model & Filter
  note: Active and reactive power controllers
  note: PLL
  note: Inputs
  Pset : Inport
  Qset : Inport  Port=2
  theta1_p : Inport  Port=3
  theta2_p : Inport  Port=4
  theta3_q : Inport  Port=5
  Add6 : Sum  Inputs=+-
  C_dc1 : powerlib/Elements/Series RLC Branch  LConnTagsString=__new0  RConnTagsString=__new0  BranchType=C  Resistance=1  Inductance=1e-3  SetiL0=off  InitialCurrent=0  Capacitance=C_dc_DVPP_3_3  Setx0=off  InitialVoltage=Vdc_n  Measurements=None
  Constant : Constant  Value=i_star_max
  Constant1 : Constant  Value=Vdc_n_DVPP_3_3
  Converter State Deviation for DVPP with DC side : Subsystem
  Current Loop : Subsystem  AncestorBlock=Library/Grid-Forming Converter Controlled by Droop Control /Current Loop
  Demux2 : Demux  Outputs=3
  G_dc1 : powerlib/Elements/Series RLC Branch  LConnTagsString=__new0  RConnTagsString=__new0  BranchType=R  Resistance=R_dc_DVPP_3_3  Inductance=1e-3  SetiL0=off  InitialCurrent=0  Capacitance=1e-6  Setx0=off  InitialVoltage=0  Measurements=None
  Gain1 : Gain  Gain=1/I_m_DVPP_3_3
  Gain10 : Gain  Gain=V_m_DVPP_3_3
  Gain16 : Gain  Gain=k_dc_DVPP_3_3
  Gain19 : Gain  Gain=2/(Vdc_n_DVPP_3_3)
  Gain3 : Gain  Gain=V_m_DVPP_3_3
  Gain4 : Gain  Gain=I_m_DVPP_3_3
  Gain5 : Gain  Gain=1/Sb_DVPP_3_3
  Gain6 : Gain  Gain=1/Sb_DVPP_3_3
  LTI System1 : cstblocks/LTI System  sys=tf(1,[tau_dc_DVPP_3_3 1])  IC=[]
  Memory10 : Memory  InitialCondition=[vabc_DVPP_3_3_0_pu(1), vabc_DVPP_3_3_0_pu(2), vabc_DVPP_3_3_0_pu(3)]
  Memory11 : Memory  InitialCondition=[iabc_DVPP_3_3_0(1), iabc_DVPP_3_3_0(2), iabc_DVPP_3_3_0(3)]
  Memory4 : Memory
  PLL : Subsystem
  "Power (dq0, Instantaneous)" : powerlib_meascontrol/Measurements/Power (dq0, Instantaneous)
      settings: SourceProductBaseCode=PS
  Power Controllers1 : Subsystem
  RL Filter Element : powerlib/Elements/Three-Phase Series RLC Branch  LConnTagsString=A|B|C  RConnTagsString=A|B|C  BranchType=RL  Resistance=R_f_DVPP_3_3  Inductance=L_f_DVPP_3_3  Capacitance=0  Measurements=Branch currents
  Reference current limitation : Subsystem
  Scope1 : Scope
  Sqrt2 : Sqrt  SaturateOnIntegerOverflow=on
  Sum2 : Sum  Inputs=+++  InputSameDT=on  SaturateOnIntegerOverflow=on  OutDataTypeStr=Inherit: Same as first input
  Three-Phase V-I Measurement : powerlib/Measurements/Three-Phase V-I Measurement  VoltageMeasurement=phase-to-ground  SetLabelV=off  LabelV=Vabc  Vpu=on  VpuLL=off  CurrentMeasurement=yes  SetLabelI=off  LabelI=Iabc  Ipu=off  Pbase=Sb_conv  Vbase=VbLV_DVPP_3_3  OutputType=Complex  PhasorSimulation=off  PSBequivalent=0
  Universal Bridge : powerlib/Power Electronics/Universal Bridge  Arms=3  SnubberResistance=1e5  SnubberCapacitance=inf  Device=Average-model based VSC  Ron=1e-3  Lon=0  ForwardVoltages="[  0  0  ]"  ForwardVoltage=0  GTOparameters=[ 10e-6 , 20e-6 ]  IGBTparameters=[ 1e-6 , 2e-6 ]  Measurements=None  Measurements_2=None  converterType=Rectifier
  Voltage Measurement : powerlib/Measurements/Voltage Measurement  PhasorSimulation=off  OutputType=Complex  PSBequivalent=0
  abc to dq1 : powerlib_meascontrol/Transformations/abc to dq0  Alignment=90 degrees behind phase A axis
  abc to dq2 : powerlib_meascontrol/Transformations/abc to dq0  Alignment=90 degrees behind phase A axis
  abc to dq3 : powerlib_meascontrol/Transformations/abc to dq0  Alignment=90 degrees behind phase A axis
  dq0 to abc : powerlib_meascontrol/Transformations/dq0 to abc  Alignment=90 degrees behind phase A axis
  d²2 : Product  InputSameDT=on  RndMeth=Zero  SaturateOnIntegerOverflow=on  OutDataTypeStr=Inherit: Same as first input
  i_dc1 : powerlib/Electrical Sources/Controlled Current Source  Initialize=off  Source_Type=DC  Amplitude=i_dc  Phase=0  Frequency=0  Measurements=None
  q²4 : Product  InputSameDT=on  RndMeth=Zero  SaturateOnIntegerOverflow=on  OutDataTypeStr=Inherit: Same as first input
  q²5 : Product  InputSameDT=on  RndMeth=Zero  SaturateOnIntegerOverflow=on  OutDataTypeStr=Inherit: Same as first input
  A : PMIOPort  Side=Right
  B : PMIOPort  Port=2  Side=Right
  C : PMIOPort  Port=3  Side=Right
  w_pll : Outport  VectorParamsAs1DForOutWhenUnconnected=off
  V : Outport  Port=2  VectorParamsAs1DForOutWhenUnconnected=off
  P : Outport  Port=3  VectorParamsAs1DForOutWhenUnconnected=off
  Theta : Outport  Port=4  VectorParamsAs1DForOutWhenUnconnected=off
  Q : Outport  Port=5  VectorParamsAs1DForOutWhenUnconnected=off
  p_des : Outport  Port=6  VectorParamsAs1DForOutWhenUnconnected=off
  i_star_dq03 : Outport  Port=7  VectorParamsAs1DForOutWhenUnconnected=off
  |i_star3_lim| : Outport  Port=8  VectorParamsAs1DForOutWhenUnconnected=off
  q_des : Outport  Port=9  VectorParamsAs1DForOutWhenUnconnected=off
  PQ_des_DVPP3 : Outport  Port=10  VectorParamsAs1DForOutWhenUnconnected=off
  wires:
  [p_des] -> p_des/1
  Memory10/1 -> [v_abc]
  [Pset] -> Power Controllers1/5(P_set)
  PLL/3(w_pll) -> [w_pll]
  PLL/2(v_dq0) -> [v_dq0]
  Demux2/2 -> q²4/1, q²4/2  "q"
  q²4/1 -> Sum2/2
  abc to dq1/1 -> "Power (dq0, Instantaneous)"/2
  Gain3/1 -> abc to dq2/1
  Reference current limitation/2(||i_star_dq0||) -> Scope1/1
  [P_abc] -> Power Controllers1/4(P_abc)
  [w_pll] -> Power Controllers1/3(w_pll)
  Demux2/1 -> d²2/1, d²2/2  "d"
  Constant1/1 -> Add6/1
  [theta_pll] -> abc to dq3/2
  Current Loop/1(v_s_ref_dq0) -> [v_s_ref_dq0]
  Gain19/1 -> Universal Bridge/1
  [Q_abc] -> Q/1
  abc to dq3/1 -> [i_dq0]
  [v_abc] -> PLL/1(v_abc)
  [w_pll] -> Current Loop/4(w_pll)
  Sqrt2/1 -> [V]
  Three-Phase V-I Measurement/2 -> Memory11/1
  Gain16/1 -> LTI System1/1
  [theta_pll] -> abc to dq2/2, abc to dq1/2
  [i_abc] -> abc to dq3/1
  "Power (dq0, Instantaneous)"/1 -> Gain5/1
  abc to dq2/1 -> "Power (dq0, Instantaneous)"/1
  Power Controllers1/2(p_des) -> [p_des]
  [Q_abc] -> Power Controllers1/1(Q_abc)
  [v_dc] -> Add6/2
  "Power (dq0, Instantaneous)"/2 -> Gain6/1
  [i_star3_lim] -> |i_star3_lim|/1
  Add6/1 -> Gain16/1
  q²5/1 -> Sum2/3
  Demux2/3 -> q²5/2, q²5/1  "0"
  dq0 to abc/1 -> Gain19/1
  Gain6/1 -> [Q_abc]
  [i_star_dq03_lim] -> i_star_dq03/1
  Gain10/1 -> dq0 to abc/1
  d²2/1 -> Sum2/1
  Current Loop/2(x_id) -> [x_id]
  [w_pll] -> w_pll/1
  [i_dq0] -> Current Loop/3(i_dq0)
  [v_abc] -> Gain3/1
  Gain5/1 -> [P_abc]
  PLL/1(theta_pll) -> [theta_pll]
  Gain1/1 -> [i_abc]
  Power Controllers1/1(i_star_dq0) -> Reference current limitation/1(i_star_dq0)
  Power Controllers1/3(q_des) -> [q_des]
  Current Loop/3(x_iq) -> [x_iq]
  Reference current limitation/3(||i_star_dq0_lim||) -> [i_star3_lim]
  [Delta_x_c] -> Power Controllers1/2(Delta x_c)
  [theta_pll] -> Theta/1
  [v_dq0] -> Current Loop/2(v_dq0)
  Three-Phase V-I Measurement/1 -> Memory10/1
  Voltage Measurement/1 -> Memory4/1
  [v_s_ref_dq0] -> Gain10/1
  Reference current limitation/1(i_star_dq0_lim) -> [i_star_dq03_lim]
  Memory11/1 -> Gain1/1
  Constant/1 -> Reference current limitation/2(i_star_max)
  [theta_pll] -> dq0 to abc/2
  Memory4/1 -> [v_dc]
  Gain4/1 -> abc to dq1/1
  [q_des] -> q_des/1
  [i_abc] -> Gain4/1
  [P_abc] -> P/1
  LTI System1/1 -> i_dc1/1
  Sum2/1 -> Sqrt2/1
  [V] -> Power Controllers1/6(|V|)
  [V] -> V/1
  [v_dq0] -> Demux2/1
  PLL/4(x_pll) -> [x_pll]
  [Qset] -> Converter State Deviation for DVPP with DC side/3(Qset)
  [x_id] -> Converter State Deviation for DVPP with DC side/4(x_id)
  [x_iq] -> Converter State Deviation for DVPP with DC side/5(x_iq)
  Converter State Deviation for DVPP with DC side/1(Delta x_c) -> [Delta_x_c]
  [Pset] -> Converter State Deviation for DVPP with DC side/2(Pset)
  [i_dq0] -> Converter State Deviation for DVPP with DC side/1(i_dq0)
  [Qset] -> Power Controllers1/7(Q_set)
  Pset/1 -> [Pset]
  Qset/1 -> [Qset]
  theta1_p/1 -> [theta1_p]
  theta2_p/1 -> [theta2_p]
  theta3_q/1 -> [theta3_q]
  [theta3_q] -> Power Controllers1/10(theta3_q)
  [theta2_p] -> Power Controllers1/9(theta2_p)
  [theta1_p] -> Power Controllers1/8(theta1_p)
  Power Controllers1/4(PQ_des_DVPP3) -> [PQ_des_DVPP3]
  [PQ_des_DVPP3] -> PQ_des_DVPP3/1
  [i_star_dq03_lim] -> Current Loop/1(i_star_dq0)
  connections:
  G_dc1/RConn1 -- C_dc1/RConn1 -- Voltage Measurement/LConn2 -- Universal Bridge/RConn2 -- i_dc1/LConn1
  Voltage Measurement/LConn1 -- Universal Bridge/RConn1 -- C_dc1/LConn1 -- i_dc1/RConn1 -- G_dc1/LConn1
  Three-Phase V-I Measurement/LConn2 -- RL Filter Element/LConn2
  RL Filter Element/RConn3 -- Universal Bridge/LConn3
  C/RConn1 -- Three-Phase V-I Measurement/RConn3
  Three-Phase V-I Measurement/LConn3 -- RL Filter Element/LConn3
  RL Filter Element/RConn2 -- Universal Bridge/LConn2
  A/RConn1 -- Three-Phase V-I Measurement/RConn1
  Three-Phase V-I Measurement/LConn1 -- RL Filter Element/LConn1
  B/RConn1 -- Three-Phase V-I Measurement/RConn2
  RL Filter Element/RConn1 -- Universal Bridge/LConn1

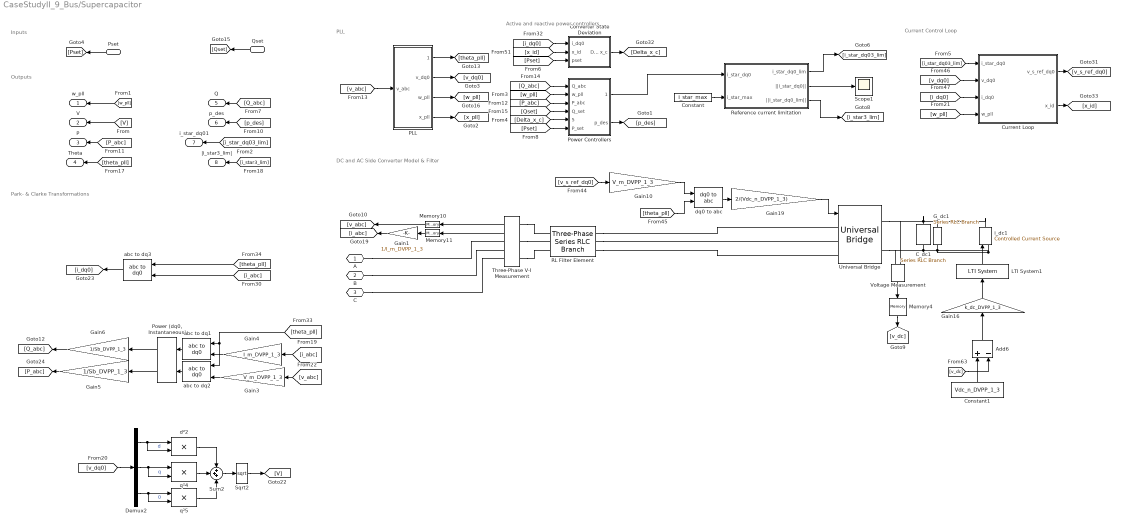
== system CaseStudyII_9_Bus/Supercapacitor ==
  note: Inputs
  note: Active and reactive power controllers
  note: PLL
  note: Outputs
  note: Current Control Loop
  note: Park- & Clarke Transformations
  note: DC and AC Side Converter Model & Filter
  Qset : Inport
  Pset : Inport  Port=2
  Add6 : Sum  Inputs=+-
  C_dc1 : powerlib/Elements/Series RLC Branch  LConnTagsString=__new0  RConnTagsString=__new0  BranchType=C  Resistance=1  Inductance=1e-3  SetiL0=off  InitialCurrent=0  Capacitance=C_dc_DVPP_1_3  Setx0=off  InitialVoltage=Vdc_n  Measurements=None
  Constant : Constant  Value=i_star_max
  Constant1 : Constant  Value=Vdc_n_DVPP_1_3
  Converter State Deviation : Subsystem
  Current Loop : Subsystem  AncestorBlock=Library/Grid-Forming Converter Controlled by Droop Control /Current Loop
  Demux2 : Demux  Outputs=3
  G_dc1 : powerlib/Elements/Series RLC Branch  LConnTagsString=__new0  RConnTagsString=__new0  BranchType=R  Resistance=R_dc_DVPP_1_3  Inductance=1e-3  SetiL0=off  InitialCurrent=0  Capacitance=1e-6  Setx0=off  InitialVoltage=0  Measurements=None
  Gain1 : Gain  Gain=1/I_m_DVPP_1_3
  Gain10 : Gain  Gain=V_m_DVPP_1_3
  Gain16 : Gain  Gain=k_dc_DVPP_1_3
  Gain19 : Gain  Gain=2/(Vdc_n_DVPP_1_3)
  Gain3 : Gain  Gain=V_m_DVPP_1_3
  Gain4 : Gain  Gain=I_m_DVPP_1_3
  Gain5 : Gain  Gain=1/Sb_DVPP_1_3
  Gain6 : Gain  Gain=1/Sb_DVPP_1_3
  LTI System1 : cstblocks/LTI System  sys=tf(1,[tau_dc_DVPP_1_3 1])  IC=[]
  Memory10 : Memory  InitialCondition=[vabc_DVPP_1_3_0_pu(1), vabc_DVPP_1_3_0_pu(2), vabc_DVPP_1_3_0_pu(3)]
  Memory11 : Memory  InitialCondition=[iabc_DVPP_1_3_0(1), iabc_DVPP_1_3_0(2), iabc_DVPP_1_3_0(3)]
  Memory4 : Memory
  PLL : Subsystem
  "Power (dq0, Instantaneous)" : powerlib_meascontrol/Measurements/Power (dq0, Instantaneous)
      settings: SourceProductBaseCode=PS
  Power Controllers : Subsystem
  RL Filter Element : powerlib/Elements/Three-Phase Series RLC Branch  LConnTagsString=A|B|C  RConnTagsString=A|B|C  BranchType=RL  Resistance=R_f_DVPP_1_3  Inductance=L_f_DVPP_1_3  Capacitance=0  Measurements=Branch currents
  Reference current limitation : Subsystem
  Scope1 : Scope
  Sqrt2 : Sqrt  SaturateOnIntegerOverflow=on
  Sum2 : Sum  Inputs=+++  InputSameDT=on  SaturateOnIntegerOverflow=on  OutDataTypeStr=Inherit: Same as first input
  Three-Phase V-I Measurement : powerlib/Measurements/Three-Phase V-I Measurement  VoltageMeasurement=phase-to-ground  SetLabelV=off  LabelV=Vabc  Vpu=on  VpuLL=off  CurrentMeasurement=yes  SetLabelI=off  LabelI=Iabc  Ipu=off  Pbase=Sb_conv  Vbase=VbLV_DVPP_1_3  OutputType=Complex  PhasorSimulation=off  PSBequivalent=0
  Universal Bridge : powerlib/Power Electronics/Universal Bridge  Arms=3  SnubberResistance=1e5  SnubberCapacitance=inf  Device=Average-model based VSC  Ron=1e-3  Lon=0  ForwardVoltages="[  0  0  ]"  ForwardVoltage=0  GTOparameters=[ 10e-6 , 20e-6 ]  IGBTparameters=[ 1e-6 , 2e-6 ]  Measurements=None  Measurements_2=None  converterType=Rectifier
  Voltage Measurement : powerlib/Measurements/Voltage Measurement  PhasorSimulation=off  OutputType=Complex  PSBequivalent=0
  abc to dq1 : powerlib_meascontrol/Transformations/abc to dq0  Alignment=90 degrees behind phase A axis
  abc to dq2 : powerlib_meascontrol/Transformations/abc to dq0  Alignment=90 degrees behind phase A axis
  abc to dq3 : powerlib_meascontrol/Transformations/abc to dq0  Alignment=90 degrees behind phase A axis
  dq0 to abc : powerlib_meascontrol/Transformations/dq0 to abc  Alignment=90 degrees behind phase A axis
  d²2 : Product  InputSameDT=on  RndMeth=Zero  SaturateOnIntegerOverflow=on  OutDataTypeStr=Inherit: Same as first input
  i_dc1 : powerlib/Electrical Sources/Controlled Current Source  Initialize=off  Source_Type=DC  Amplitude=i_dc  Phase=0  Frequency=0  Measurements=None
  q²4 : Product  InputSameDT=on  RndMeth=Zero  SaturateOnIntegerOverflow=on  OutDataTypeStr=Inherit: Same as first input
  q²5 : Product  InputSameDT=on  RndMeth=Zero  SaturateOnIntegerOverflow=on  OutDataTypeStr=Inherit: Same as first input
  A : PMIOPort  Side=Right
  B : PMIOPort  Port=2  Side=Right
  C : PMIOPort  Port=3  Side=Right
  w_pll : Outport  VectorParamsAs1DForOutWhenUnconnected=off
  V : Outport  Port=2  VectorParamsAs1DForOutWhenUnconnected=off
  P : Outport  Port=3  VectorParamsAs1DForOutWhenUnconnected=off
  Theta : Outport  Port=4  VectorParamsAs1DForOutWhenUnconnected=off
  Q : Outport  Port=5  VectorParamsAs1DForOutWhenUnconnected=off
  p_des : Outport  Port=6  VectorParamsAs1DForOutWhenUnconnected=off
  i_star_dq01 : Outport  Port=7  VectorParamsAs1DForOutWhenUnconnected=off
  |i_star3_lim| : Outport  Port=8  VectorParamsAs1DForOutWhenUnconnected=off
  wires:
  PLL/4(x_pll) -> [x_pll]
  [v_abc] -> PLL/1(v_abc)
  [i_star_dq03_lim] -> i_star_dq01/1
  PLL/2(v_dq0) -> [v_dq0]
  [p_des] -> p_des/1
  PLL/1(theta_pll) -> [theta_pll]
  PLL/3(w_pll) -> [w_pll]
  [V] -> V/1
  [w_pll] -> w_pll/1
  [theta_pll] -> Theta/1
  Power Controllers/2(p_des) -> [p_des]
  [Q_abc] -> Q/1
  Qset/1 -> [Qset]
  [P_abc] -> P/1
  Constant/1 -> Reference current limitation/2(i_star_max)
  Reference current limitation/2(||i_star_dq0||) -> Scope1/1
  [i_star3_lim] -> |i_star3_lim|/1
  [w_pll] -> Current Loop/4(w_pll)
  [i_dq0] -> Current Loop/3(i_dq0)
  Reference current limitation/1(i_star_dq0_lim) -> [i_star_dq03_lim]
  [v_dq0] -> Current Loop/2(v_dq0)
  [v_dq0] -> Demux2/1
  Sum2/1 -> Sqrt2/1
  [i_abc] -> Gain4/1
  Demux2/3 -> q²5/2, q²5/1  "0"
  Gain1/1 -> [i_abc]
  Memory11/1 -> Gain1/1
  Demux2/1 -> d²2/1, d²2/2  "d"
  Three-Phase V-I Measurement/2 -> Memory11/1
  abc to dq1/1 -> "Power (dq0, Instantaneous)"/2
  Three-Phase V-I Measurement/1 -> Memory10/1
  Gain5/1 -> [P_abc]
  Gain4/1 -> abc to dq1/1
  Gain3/1 -> abc to dq2/1
  q²4/1 -> Sum2/2
  Gain6/1 -> [Q_abc]
  Gain19/1 -> Universal Bridge/1
  Add6/1 -> Gain16/1
  LTI System1/1 -> i_dc1/1
  [v_abc] -> Gain3/1
  [theta_pll] -> abc to dq3/2
  abc to dq3/1 -> [i_dq0]
  Voltage Measurement/1 -> Memory4/1
  d²2/1 -> Sum2/1
  [theta_pll] -> abc to dq2/2, abc to dq1/2
  dq0 to abc/1 -> Gain19/1
  Memory10/1 -> [v_abc]
  "Power (dq0, Instantaneous)"/2 -> Gain6/1
  Sqrt2/1 -> [V]
  "Power (dq0, Instantaneous)"/1 -> Gain5/1
  Demux2/2 -> q²4/1, q²4/2  "q"
  [v_dc] -> Add6/2
  q²5/1 -> Sum2/3
  abc to dq2/1 -> "Power (dq0, Instantaneous)"/1
  Memory4/1 -> [v_dc]
  Gain10/1 -> dq0 to abc/1
  [theta_pll] -> dq0 to abc/2
  [i_abc] -> abc to dq3/1
  [v_s_ref_dq0] -> Gain10/1
  Gain16/1 -> LTI System1/1
  Constant1/1 -> Add6/1
  Current Loop/2(x_id) -> [x_id]
  Current Loop/1(v_s_ref_dq0) -> [v_s_ref_dq0]
  [P_abc] -> Power Controllers/3(P_abc)
  [w_pll] -> Power Controllers/2(w_pll)
  [Delta_x_c] -> Power Controllers/5(Delta x_c)
  [Q_abc] -> Power Controllers/1(Q_abc)
  [Qset] -> Power Controllers/4(Q_set)
  Reference current limitation/3(||i_star_dq0_lim||) -> [i_star3_lim]
  [i_star_dq03_lim] -> Current Loop/1(i_star_dq0)
  Power Controllers/1(i_star_dq0) -> Reference current limitation/1(i_star_dq0)
  [Pset] -> Converter State Deviation/3(pset)
  [x_id] -> Converter State Deviation/2(x_id)
  [i_dq0] -> Converter State Deviation/1(i_dq0)
  Converter State Deviation/1(Delta x_c) -> [Delta_x_c]
  [Pset] -> Power Controllers/6(P_set)
  Pset/1 -> [Pset]
  connections:
  i_dc1/LConn1 -- G_dc1/RConn1 -- Voltage Measurement/LConn2 -- Universal Bridge/RConn2 -- C_dc1/RConn1
  i_dc1/RConn1 -- Universal Bridge/RConn1 -- Voltage Measurement/LConn1 -- C_dc1/LConn1 -- G_dc1/LConn1
  Three-Phase V-I Measurement/LConn2 -- RL Filter Element/LConn2
  RL Filter Element/RConn3 -- Universal Bridge/LConn3
  B/RConn1 -- Three-Phase V-I Measurement/RConn2
  C/RConn1 -- Three-Phase V-I Measurement/RConn3
  Three-Phase V-I Measurement/LConn1 -- RL Filter Element/LConn1
  RL Filter Element/RConn2 -- Universal Bridge/LConn2
  A/RConn1 -- Three-Phase V-I Measurement/RConn1
  Three-Phase V-I Measurement/LConn3 -- RL Filter Element/LConn3
  RL Filter Element/RConn1 -- Universal Bridge/LConn1
